simulink model "Linearity_Test"  (R2018b)
settings: Solver=VariableStepAuto  StartTime=0.0  StopTime=10.0  RelTol=1e-3
settings Model: Creator=hp  LastModifiedBy=hp

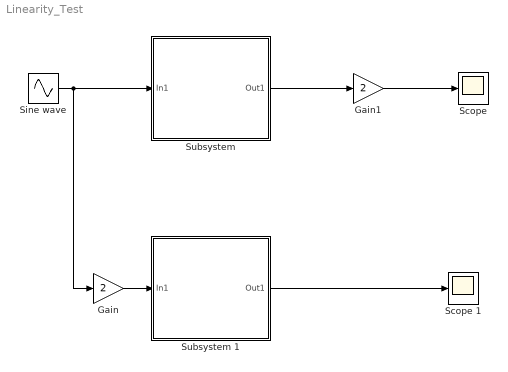
== system Linearity_Test ==
  Gain : Gain  Gain=2
  Gain1 : Gain  Gain=2
  "Scope " : Scope
  Scope 1 : Scope
  Sine wave : Sin  SampleTime=0
  "Subsystem " : Subsystem
  Subsystem 1 : Subsystem
  wires:
  "Subsystem "/1(Out1) -> Gain1/1
  Gain1/1 -> "Scope "/1
  Gain/1 -> Subsystem 1/1(In1)
  Sine wave/1 -> Gain/1, "Subsystem "/1(In1)
  Subsystem 1/1(Out1) -> Scope 1/1

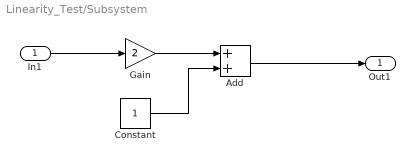
== system Linearity_Test/Subsystem  ==
  In1 : Inport
  "Add " : Sum
  "Constant " : Constant
  "Gain " : Gain  Gain=2
  Out1 : Outport
  wires:
  "Constant "/1 -> "Add "/2
  "Add "/1 -> Out1/1
  In1/1 -> "Gain "/1
  "Gain "/1 -> "Add "/1

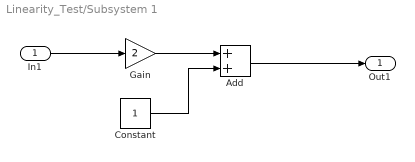
== system Linearity_Test/Subsystem 1 ==
  In1 : Inport
  "Add " : Sum
  "Constant " : Constant
  "Gain " : Gain  Gain=2
  Out1 : Outport
  wires:
  "Constant "/1 -> "Add "/2
  "Add "/1 -> Out1/1
  In1/1 -> "Gain "/1
  "Gain "/1 -> "Add "/1
